simulink model "DCC_DTC_v2_copy_properMotorParameters"  (R2023b)
settings: Solver=FixedStepDiscrete  StartTime=0.0  StopTime=0.4  MaxStep=1e-  RelTol=1e-6
undefined symbols (not defined in the file): DiscIntNeverNeededParam
libraries: spsDCVoltageSourceLib x1, spsGroundLib x1, spsPermanentMagnetSynchronousMachineLib x1, simulink x1, spsThreePhaseVIMeasurementLib x1, spsUniversalBridgeLib x1, sps_lib x1
settings Model: Creator=rainy  LastModifiedBy=rainy
settings DataIOCC: ReturnWorkspaceOutputs=off

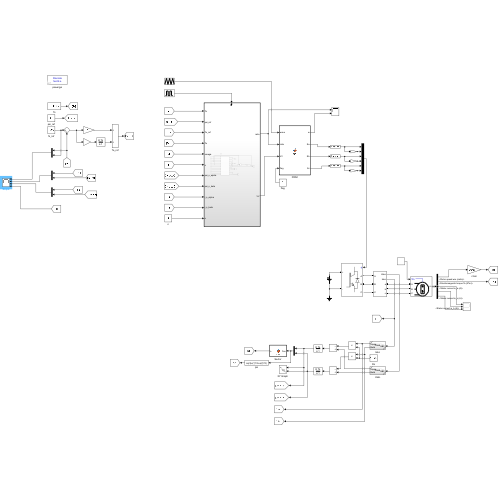
[thumbnail: Simulink's stored preview of the top-level diagram]
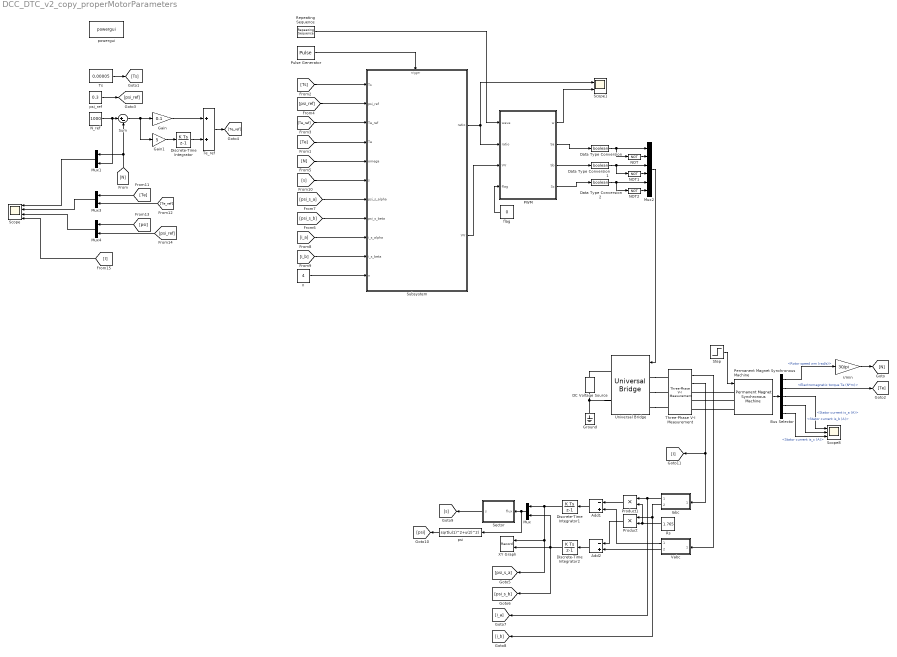
== system DCC_DTC_v2_copy_properMotorParameters ==
  Add1 : Sum  Inputs=-+
  Add2 : Sum  Inputs=-+
  Bus Selector : BusSelector  OutputSignals=Rotor speed wm (rad/s),Electromagnetic torque Te (N*m),Stator current is_a (A),Stator current is_b (A),Stator current is_c (A)
  DC Voltage Source : spsDCVoltageSourceLib/DC Voltage Source  Amplitude=300  Measurements=Voltage
  Data Type Conversion : DataTypeConversion  OutDataTypeStr=boolean  SaturateOnIntegerOverflow=off  RndMeth=Floor
  Data Type Conversion1 : DataTypeConversion  OutDataTypeStr=boolean  SaturateOnIntegerOverflow=off  RndMeth=Floor
  Data Type Conversion2 : DataTypeConversion  OutDataTypeStr=boolean  SaturateOnIntegerOverflow=off  RndMeth=Floor
  Discrete-Time Integrator : DiscreteIntegrator  SampleTime=-1  ICPrevOutput=DiscIntNeverNeededParam  ICPrevScaledInput=DiscIntNeverNeededParam
  Discrete-Time Integrator1 : DiscreteIntegrator  SampleTime=-1  ICPrevOutput=DiscIntNeverNeededParam  ICPrevScaledInput=DiscIntNeverNeededParam
  Discrete-Time Integrator2 : DiscreteIntegrator  SampleTime=-1  ICPrevOutput=DiscIntNeverNeededParam  ICPrevScaledInput=DiscIntNeverNeededParam
  Gain : Gain  Gain=0.1
  Gain1 : Gain  Gain=5
  Ground : spsGroundLib/Ground  LConnTagsString=a
  Iabc : Subsystem  ReferencedSubsystem=Clark
  Mux{,1,3..4} (4 alike) : Mux  Inputs=2
  Mux2 : Mux  Inputs=6
  NOT : Logic  Operator=NOT  IconShape=distinctive  AllPortsSameDT=off  OutDataTypeStr=boolean
  NOT1 : Logic  Operator=NOT  IconShape=distinctive  AllPortsSameDT=off  OutDataTypeStr=boolean
  NOT2 : Logic  Operator=NOT  IconShape=distinctive  AllPortsSameDT=off  OutDataTypeStr=boolean
  N_ref : Constant  Value=1000
  PWM : MATLAB Function  TreatAsAtomicUnit=on
  Permanent Magnet Synchronous Machine : spsPermanentMagnetSynchronousMachineLib/Permanent Magnet Synchronous Machine  NbPhases=3  FluxDistribution=Sinusoidal  RotorType=Salient-pole  MechanicalLoad=Torque Tm  PresetModel="02:  1.7 Nm 300 Vdc 3750 RPM - 1.7 Nm"  ShowDetailedParameters=on  MeasurementBus=off  Resistance=4.765  Inductance=8.5e-3  dqInductances=[0.0133 0.0147]  La=0.014  MachineConstant=Flux linkage established by magnets (V.s)  Flux=0.1848  VoltageCst=67.1831  TorqueCst=0.5556  Flat=120  Mechanical=[0.0001051 4.047e-05 2 0]  PolePairs=2  InitialConditions=[0 0 0 0]  InitialConditions5ph=[0 0 0 0 0 0]  RefAngle=Aligned with phase A axis (original Park)  IterativeDiscreteModel=Trapezoidal non iterative  TsBlock=-1  TsPowergui=0
  Product : Product
  Product1 : Product
  Pulse Generator : DiscretePulseGenerator  PulseType=Time based  Period=0.00005
  Repeating Sequence : simulink/Sources/Repeating Sequence  rep_seq_t=[0 0.000025 0.00005]  rep_seq_y=[0 1 0]
  Rs : Constant  Value=1.765
  Scope : Scope  NumInputPorts=4
  Scope1 : Scope  NumInputPorts=2
  Scope8 : Scope  NumInputPorts=3
  Sector : MATLAB Function  TreatAsAtomicUnit=on
  Step : Step  Time=0.2  SampleTime=0
  Subsystem : Subsystem
  Sum : Sum  Inputs=|+-
  Te_ref : Sum
  Three-Phase V-I Measurement : spsThreePhaseVIMeasurementLib/Three-Phase V-I Measurement  VoltageMeasurement=phase-to-ground  SetLabelV=off  LabelV=Vabc  Vpu=off  VpuLL=off  CurrentMeasurement=yes  SetLabelI=off  LabelI=Iabc  Ipu=off  Pbase=100e6  Vbase=500e3  OutputType=Complex  PhasorSimulation=off  PSBequivalent=0
  Ts : Constant  Value=0.00005
  Universal Bridge : spsUniversalBridgeLib/Universal Bridge  Arms=3  SnubberResistance=1e5  SnubberCapacitance=inf  Device=IGBT / Diodes  Ron=1e-3  Lon=0  ForwardVoltages="[  0  0  ]"  ForwardVoltage=0  GTOparameters=[ 10e-6 , 20e-6 ]  IGBTparameters=[ 1e-6 , 2e-6 ]  Measurements=None  Measurements_2=None  converterType=Rectifier
  Vabc : Subsystem  ReferencedSubsystem=Clark
  XY Graph : Record  FileSettingsInternal="{\"entries\":[{\"content\":{\"excelSettings\":{\"content\":{},\"type\":\"Streamout.ExcelSettings\"}},\"type\":\"Streamout.FileSettingStorage\",\"uuid\":\"\"}],\"packageUris\":[\"http:\\/\\/schema.mathworks.com\\/mf0\\/streamout_blocks\\/R2020a\"],\"version\":\"1.0\"}"  Layout=[1 1]  SignalsInternal="{\"entries\":[{\"content\":{\"signals\":[{\"content\":{\"blockPath\":[],\"dimensions\":[1],\"domain\":\"\",\"lineColor\":\"#a2142f\",\"plots\":[1],\"port\":1,\"sid\":[\"\"],\"signalID\":12404,\"signalName\":\"Discrete-Time\\nIntegrator1\"},\"type\":\"RecordBlkView.Signal\",\"uuid\":\"\"},{\"content\":{\"blockPath\":[],\"dimensions\":[1],\"domain\":\"\",\"lineColor\":\"#139fff\",\"plots\":[1],\"port\":2,\"sid\":[\"\"],\"signalID\":12408,\"signalName\":\"Discrete-Time\\nIntegrator2\"},\"type\":\"RecordBlkView.Signal\",\"uuid\":\"\"}]},\"type\":\"RecordBlkView.InputSignals\",\"uuid\":\"\"}],\"packageUris\":[\"http:\\/\\/schema.mathworks.com\\/mf0\\/streamout_blocks\\/R2020a\"],\"version\":\"1.0\"}"  VisualizationBindings="{\"xyplotplugin\":{\"info\":[{\"series\":[{\"bindingParametersList\":[{\"parameter\":\"X-Axis\",\"signalID\":12404,\"signalName\":\"Discrete-Time\\nIntegrator1\"},{\"parameter\":\"Y-Axis\",\"signalID\":12408,\"signalName\":\"Discrete-Time\\nIntegrator2\"}],\"seriesID\":32890}],\"subplotID\":1}]}}"  CompatibilityTag=XY  st=-1
  flag : Constant  Value=0
  n : Constant  Value=4
  powergui : sps_lib/powergui  Priority=1  SimulationMode=Discrete  SampleTime=5e-6  frequency=60  Iterations=50  frequencyindice=0  Pbase=100e6  ErrMax=1e-4  UnitsV=kV  UnitsW=MW  buscounter=0  FunctionMessages=off  echomessages=off  EnableUseOfTLC=off  CurrentSourceSwitches=off  DisableSnubberDevices=off  DisableRonSwitches=off  DisableVfSwitches=off  DisplayEquations=off  AutomaticDiscreteSolvers=off  SolverType=Tustin/Backward Euler (TBE)  Interpol=off  ExternalGateDelay=off  methode=off  Ts=100  x0status=blocks  SPID=on  SwTol=0  HookPort=off  NonlinearTolerance=1e-4  nMaxIteration=100  ContinueOnMaxIteration=off  RestoreLinks=warning  ResistiveCurrentMeasurement=off  Frange=[0:2:500]  Ylog=off  Xlog=on  ShowGrid=off  save=off  variable=ZData  structure=0  ZoomFFT=off  StartTime=0.0  cycles=1  DisplayStyle=1  fundamental=60  FreqAxis=off  MaxFrequency=1000  frequencyindicesteady=1  RmsSteady=1  display=off
  psi : Fcn  Expr=sqrt(u(1)^2+u(2)^2)
  psi_ref : Constant  Value=0.3
  r/min : Gain  Gain=30/pi
  wires:
  N_ref/1 -> Mux1/2, Sum/1
  Sum/1 -> Gain/1, Gain1/1
  Gain1/1 -> Discrete-Time Integrator/1
  Gain/1 -> Te_ref/1
  Permanent Magnet Synchronous Machine/1 -> Bus Selector/1
  Bus Selector/1 -> r/min/1  "<Rotor speed wm (rad/s)>"
  r/min/1 -> [N]
  [N] -> Sum/2, Mux1/1
  NOT1/1 -> Mux2/4
  Data Type Conversion2/1 -> NOT2/1, Mux2/5
  NOT2/1 -> Mux2/6
  Data Type Conversion/1 -> NOT/1, Mux2/1
  NOT/1 -> Mux2/2
  Data Type Conversion1/1 -> NOT1/1, Mux2/3
  Iabc/1 -> [i_a], Product1/1
  Iabc/2 -> [i_b], Product/1
  Rs/1 -> Product/2, Product1/2
  Product1/1 -> Add1/1
  Vabc/1 -> Add1/2
  Product/1 -> Add2/1
  Vabc/2 -> Add2/2
  Add2/1 -> Discrete-Time Integrator2/1
  Add1/1 -> Discrete-Time Integrator1/1
  Ts/1 -> [Ts]
  Discrete-Time Integrator1/1 -> Mux/1, [psi_s_a], XY Graph/1
  Discrete-Time Integrator2/1 -> [psi_s_b], XY Graph/2, Mux/2
  Mux/1 -> psi/1, Sector/1(flux)
  Bus Selector/2 -> [Te]  "<Electromagnetic torque Te (N*m)>"
  [Te] -> Subsystem/4(Te)
  Three-Phase V-I Measurement/2 -> [I], Iabc/1
  Three-Phase V-I Measurement/1 -> Vabc/1
  Discrete-Time Integrator/1 -> Te_ref/2
  psi_ref/1 -> [psi_ref]
  PWM/4(Sc) -> Data Type Conversion2/1
  PWM/3(Sb) -> Data Type Conversion1/1
  PWM/2(Sa) -> Data Type Conversion/1
  [Ts] -> Subsystem/1(Ts)
  [psi_ref] -> Subsystem/2(psi_ref)
  Repeating Sequence/1 -> PWM/1(wave)
  Pulse Generator/1 -> Subsystem/Trigger
  n/1 -> Subsystem/11(n)
  flag/1 -> PWM/4(flag)
  Bus Selector/3 -> Scope8/1  "<Stator current is_a (A)>"
  Bus Selector/4 -> Scope8/2  "<Stator current is_b (A)>"
  Bus Selector/5 -> Scope8/3  "<Stator current is_c (A)>"
  Step/1 -> Permanent Magnet Synchronous Machine/1
  Subsystem/1(ratio) -> Scope1/1, PWM/2(ratio)
  Subsystem/2(VV) -> PWM/3(VV)
  Te_ref/1 -> [Te_ref]
  [Te_ref] -> Subsystem/3(Te_ref)
  [N] -> Subsystem/5(omega)
  [i_a] -> Subsystem/9(i_s_alpha)
  [i_b] -> Subsystem/10(i_s_beta)
  [psi_s_b] -> Subsystem/8(psi_s_beta)
  [psi_s_a] -> Subsystem/7(psi_s_alpha)
  Sector/1(s) -> [s]
  [s] -> Subsystem/6(s)
  PWM/1(w) -> Scope1/2
  psi/1 -> [psi]
  Mux1/1 -> Scope/1
  Mux3/1 -> Scope/2
  Mux4/1 -> Scope/3
  [I] -> Scope/4
  [Te] -> Mux3/1
  [psi] -> Mux4/1
  [Te_ref] -> Mux3/2
  [psi_ref] -> Mux4/2
  Mux2/1 -> Universal Bridge/1
  connections:
  Universal Bridge/RConn2 -- Ground/LConn1 -- DC Voltage Source/LConn1
  Permanent Magnet Synchronous Machine/LConn2 -- Three-Phase V-I Measurement/RConn2
  Permanent Magnet Synchronous Machine/LConn1 -- Three-Phase V-I Measurement/RConn1
  Universal Bridge/LConn3 -- Three-Phase V-I Measurement/LConn3
  Universal Bridge/LConn1 -- Three-Phase V-I Measurement/LConn1
  Universal Bridge/LConn2 -- Three-Phase V-I Measurement/LConn2
  DC Voltage Source/RConn1 -- Universal Bridge/RConn1
  Permanent Magnet Synchronous Machine/LConn3 -- Three-Phase V-I Measurement/RConn3

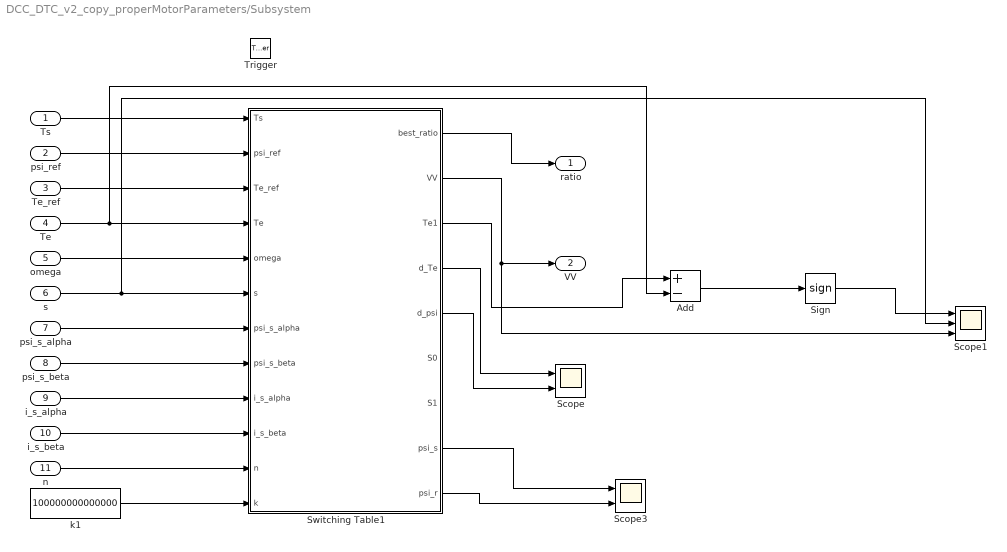
== system DCC_DTC_v2_copy_properMotorParameters/Subsystem ==
  Ts : Inport
  psi_ref : Inport  Port=2
  Te_ref : Inport  Port=3
  Te : Inport  Port=4
  omega : Inport  Port=5
  s : Inport  Port=6
  psi_s_alpha : Inport  Port=7
  psi_s_beta : Inport  Port=8
  i_s_alpha : Inport  Port=9
  i_s_beta : Inport  Port=10
  n : Inport  Port=11
  Trigger : TriggerPort  VariantControl=(inherit)  PortDimensions=1
  Add : Sum  Inputs=+-
  Scope : Scope  NumInputPorts=2
  Scope1 : Scope  NumInputPorts=3
  Scope3 : Scope  NumInputPorts=2
  Sign : Signum
  Switching Table1 : MATLAB Function  TreatAsAtomicUnit=on
  k1 : Constant  Value=100000000000000
  ratio : Outport
  VV : Outport  Port=2
  wires:
  Ts/1 -> Switching Table1/1(Ts)
  psi_ref/1 -> Switching Table1/2(psi_ref)
  Te_ref/1 -> Switching Table1/3(Te_ref)
  Te/1 -> Add/2, Switching Table1/4(Te)
  omega/1 -> Switching Table1/5(omega)
  s/1 -> Scope1/2, Switching Table1/6(s)
  psi_s_alpha/1 -> Switching Table1/7(psi_s_alpha)
  psi_s_beta/1 -> Switching Table1/8(psi_s_beta)
  i_s_alpha/1 -> Switching Table1/9(i_s_alpha)
  i_s_beta/1 -> Switching Table1/10(i_s_beta)
  Switching Table1/1(best_ratio) -> ratio/1
  k1/1 -> Switching Table1/12(k)
  n/1 -> Switching Table1/11(n)
  Switching Table1/2(VV) -> Scope1/3, VV/1
  Switching Table1/4(d_Te) -> Scope/1
  Switching Table1/5(d_psi) -> Scope/2
  Switching Table1/3(Te1) -> Add/1
  Switching Table1/9(psi_r) -> Scope3/2
  Switching Table1/8(psi_s) -> Scope3/1
  Add/1 -> Sign/1
  Sign/1 -> Scope1/1

== matlab function DCC_DTC_v2_copy_properMotorParameters/Subsystem/Switching Table1 ==
  data: best_ratio output; Ts input; psi_ref input; Te_ref input; Te input; VV output; Te1 output; omega input; s input; psi_s_alpha input; psi_s_beta input; i_s_alpha input; i_s_beta input; n input; k input; d_Te output; d_psi output; S0 output; S1 output; psi_s output; psi_r output
function [best_ratio, VV, Te1, d_Te, d_psi, S0, S1, psi_s, psi_r]= fcn(Ts, psi_ref, Te_ref, Te, omega, s, psi_s_alpha, psi_s_beta, i_s_alpha, i_s_beta, n, k)

% 给定的参数值
P = 4; % 极对数
R_s = 1.2; % 定子电阻
R_r = 1.2; % 转子电阻
L_m = 0.008; % 磁链互感
L_s = 0.0085; % 定子电感
L_r = 0.0085; % 转子电感
sigma = 1-L_m^2/(L_s*L_r);
V = 311;

psi_s = psi_s_alpha + 1i*psi_s_beta;
i_s = i_s_alpha + 1i*i_s_beta;
psi_r = L_r/L_m*psi_s + i_s*(L_m - L_s*L_r/L_m);


% 计算 S0
S0 = 1.5 * P/2 * L_m/(sigma * L_s * L_r) * ...
    ( ...
    -(R_s/(sigma*L_s) + R_r/(sigma*L_r))*imag(psi_r'*psi_s) - omega*real(psi_r'*psi_s) ...
    );

Te1 = Te + Ts*S0;
psi = sqrt(psi_s_alpha^2 +psi_s_beta^2);

if(Te_ref > Te)
    if(psi_ref > psi)
        VV = s+1;
    else
        VV = s+2;
    end
else
    if(psi_ref > psi)
        VV = s-1;
    else
        VV = s-2;
    end
end

if(VV < 1)
    VV = VV+6;
end
if(VV > 6)
    VV = VV-6;
end

V_k = cos(pi/6*(VV-1))*V + 1i*sin(pi/6*(VV-1))*V;
S1 = S0 + 1.5*P/2 * L_m/(sigma*L_s*L_r) * imag(psi_r'*V_k);
S2 = 1.5*P/2 * L_m/(sigma*L_s*L_r) * imag(psi_r'*V_k);

g_min = 200000;
best_ratio = 1;

d_Te = 0;
d_psi = 0;

for i=1:n+1
    ratio = (i-1)*1/n;

    Te1_ = Te + Ts*ratio*S1 + Ts*(1-ratio)*S0;
    psi_s1 = psi_s + Ts*ratio*V_k - R_s*Ts*ratio*i_s;
    
    d_Te = abs(Te_ref - Te1_);
    d_psi = k*abs(psi_ref - abs(psi_s1));

    g = d_Te + d_psi;

    if(g < g_min)
        g_min = g;
        best_ratio =ratio;
    end
end

[d_Te d_psi best_ratio]
[Te_ref Te1 Te Ts*S0 Ts*S1 Ts*S2]

== matlab function DCC_DTC_v2_copy_properMotorParameters/Sector ==
  data: flux input; s output
function s = fcn(flux)

% 将\psi_{\aplha}和\psi_{\beta}分解为三相
a1 = flux(1);
b1 = flux(1)*(-0.5) + sqrt(3)/2*flux(2);
c1 = flux(1)*(-0.5) - sqrt(3)/2*flux(2);

% a1 > 0，有扇区126
% b1 > 0，有扇区234
% c1 > 0，有扇区456
% n为a1 b1 c1中>0的个数，0 < n < 3
% 
% a b c | s
%-------|---
% 1 1 0 | 2
% 1 0 1 | 6
% 1 0 0 | 1
% 0 1 1 | 4
% 0 1 0 | 3
% 0 0 1 | 5

if(flux(2) == 0)
    N = 4;
else
    if(a1 > 0)
        a = 1;
    else
        a = 0;
    end
    
    if(b1 > 0)
        b = 1;
    else
        b = 0;
    end
    
    if(c1 > 0)
        c = 1;
    else
        c = 0;
    end
    
    N = 4*a+2*b+c;
end

% if(N==0 || N==7)
%     N = 4;
% end

Sector_table=[5 3 4 1 6 2];

s = Sector_table(N);

== matlab function DCC_DTC_v2_copy_properMotorParameters/PWM ==
  data: w output; wave input; ratio input; VV input; Sa output; Sb output; Sc output; flag input
function [w, Sa, Sb, Sc] = fcn(wave, ratio, VV, flag)

sw = [1 0 0; 1 1 0; 0 1 0; 0 1 1; 0 0 1; 1 0 1];

if(VV<1 || VV>6)
    VV = 1;
end

if(wave >= 1 - ratio || flag == 0)
    Sa= sw(VV, 1);
    Sb= sw(VV, 2);
    Sc= sw(VV, 3);
    w = 1;
else
    Sa = 0;
    Sb = 0;
    Sc = 0;
    w = 0;
end
